simulink model "latihan2_"  (R2023a)
settings: Solver=VariableStepAuto  StartTime=0.0  StopTime=10.0  RelTol=1e-3
values from neighbouring files (symbols this model uses):
  ts1 = 0.2    [sampling_error.m]
  ts2 = 0.5    [sampling_error.m]
settings Model: Creator=User  LastModifiedBy=User

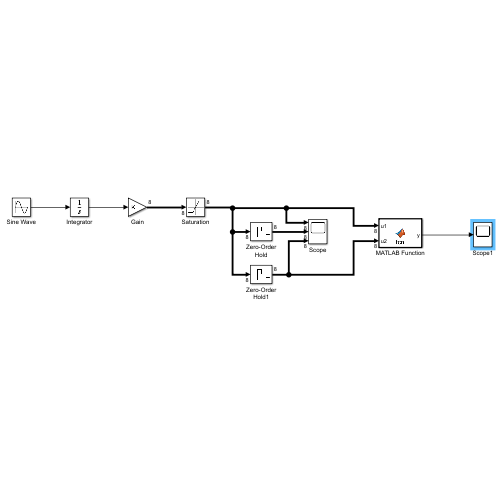
[thumbnail: Simulink's stored preview of the top-level diagram]
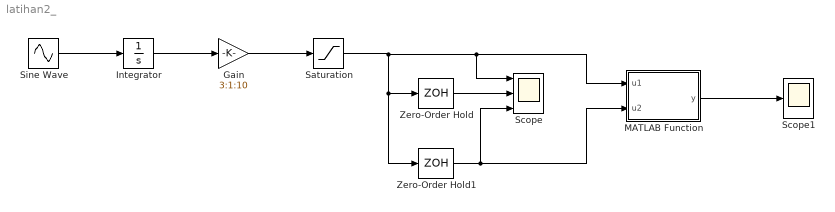
== system latihan2_ ==
  Gain : Gain  Gain=3:1:10
  Integrator : Integrator
  MATLAB Function : MATLAB Function  TreatAsAtomicUnit=on
  Saturation : Saturate
  Scope : Scope  NumInputPorts=3
  Scope1 : Scope
  Sine Wave : Sin  Amplitude=5  Frequency=5  SampleTime=0
  Zero-Order Hold : ZeroOrderHold  SampleTime=ts1
  Zero-Order Hold1 : ZeroOrderHold  SampleTime=ts2
  wires:
  Sine Wave/1 -> Integrator/1
  Integrator/1 -> Gain/1
  Gain/1 -> Saturation/1
  Saturation/1 -> Zero-Order Hold1/1, Zero-Order Hold/1, MATLAB Function/1(u1), Scope/1
  Zero-Order Hold/1 -> Scope/2
  Zero-Order Hold1/1 -> MATLAB Function/2(u2), Scope/3
  MATLAB Function/1(y) -> Scope1/1

== matlab function latihan2_/MATLAB Function ==
  data: u1 input; y output; u2 input
function y = fcn(u1, u2)

y = sampling_error(u1,u2);
